simulink model "Experiment4_DOB_model2"  (R2012b)
settings: Solver=ode3  SolverMode=SingleTasking  StartTime=0.0  StopTime=5  FixedStep=0.002  RelTol=1e-3
values from neighbouring files (symbols this model uses):
  exp_A_DOB = 1    [model_DOB.mat]
  exp_model = 1    [model_ref.mat]
  exp_model_input = 1    [model_input.mat]
undefined symbols (not defined in the file or in its folder): K0, Kd, Ki, Kp, Plant_K, Plant_T1, Plant_T2, Q_T, T1, T2
libraries: simulink x4
settings Model: Creator=taoyi  LastModifiedBy=Administrator
settings DataIOCC: SignalLoggingSaveFormat=ModelDataLogs
settings OptimizationCC: BlockReduction=off  BooleanDataType=off
settings DebuggingCC: SaveWithParameterizedLinksMsg=none  SignalResolutionControl=TryResolveAllWithWarning  SolverPrmCheckMsg=none  MultiTaskDSMMsg=warning  MultiTaskCondExecSysMsg=none  StrictBusMsg=None
settings HardwareCC: TargetUnknown=on
settings RTWCC: IncludeERTFirstTime=on

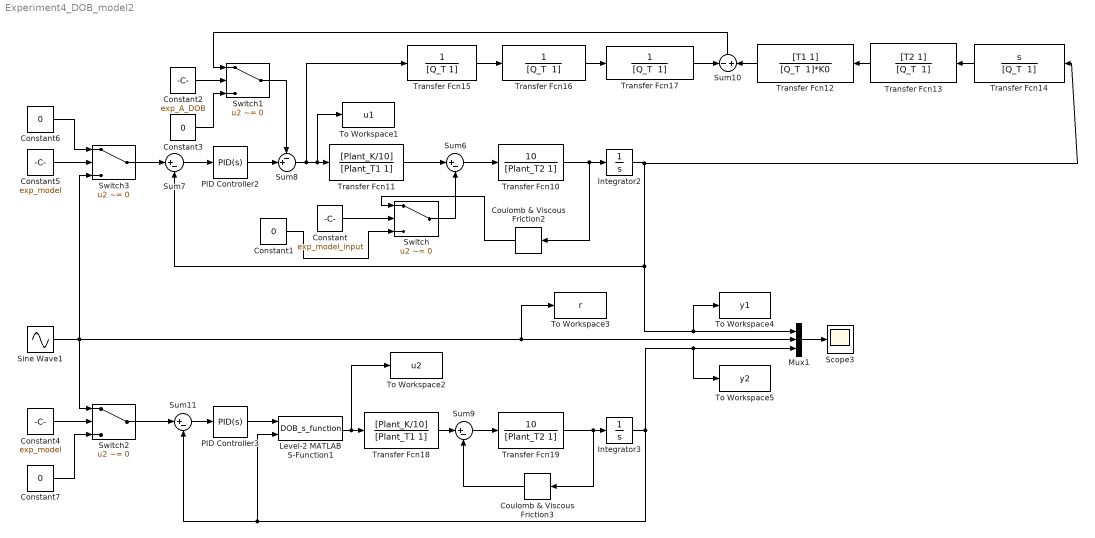
== system Experiment4_DOB_model2 ==
  Constant : Constant  Value=exp_model_input
  Constant{1,3,6..7} (4 alike) : Constant  Value=0
  Constant2 : Constant  Value=exp_A_DOB
  Constant4 : Constant  Value=exp_model
  Constant5 : Constant  Value=exp_model
  Coulomb & Viscous Friction2 : simulink/Discontinuities/Coulomb & Viscous Friction  offset=[20]  gain=0.3
  Coulomb & Viscous Friction3 : simulink/Discontinuities/Coulomb & Viscous Friction  offset=[20]  gain=0.3
  Integrator2 : Integrator
  Integrator3 : Integrator
  Level-2 MATLAB S-Function1 : M-S-Function  FunctionName=DOB_s_function  Parameters=K0,T1,T2,Q_T
  Mux1 : Mux  Inputs=3
  PID Controller2 : simulink/Continuous/PID Controller  Controller=PID  TimeDomain=Continuous-time  SampleTime=1  IntegratorMethod=Forward Euler  FilterMethod=Forward Euler  Form=Parallel  P=Kp  I=Ki  D=Kd  N=100  InitialConditionSource=internal  InitialConditionForIntegrator=0  InitialConditionForFilter=0  ExternalReset=none  LimitOutput=off  UpperSaturationLimit=inf  LowerSaturationLimit=-inf  LinearizeAsGain=on  AntiWindupMode=none  Kb=1  TrackingMode=off  Kt=1  PParamMin=[]  PParamMax=[]  IParamMin=[]  IParamMax=[]  DParamMin=[]  DParamMax=[]  NParamMin=[]  NParamMax=[]  KbParamMin=[]  KbParamMax=[]  KtParamMin=[]  KtParamMax=[]  POutMin=[]  POutMax=[]  IOutMin=[]  IOutMax=[]  DOutMin=[]  DOutMax=[]  NOutMin=[]  NOutMax=[]  KbOutMin=[]  KbOutMax=[]  KtOutMin=[]  KtOutMax=[]  IntegratorOutMin=[]  IntegratorOutMax=[]  FilterOutMin=[]  FilterOutMax=[]  SumOutMin=[]  SumOutMax=[]  SumI1OutMin=[]  SumI1OutMax=[]  SumI2OutMin=[]  SumI2OutMax=[]  SumI3OutMin=[]  SumI3OutMax=[]  SumDOutMin=[]  SumDOutMax=[]  SaturationOutMin=[]  SaturationOutMax=[]  IntegratorContinuousStateAttributes=''  IntegratorStateMustResolveToSignalObject=off  IntegratorRTWStateStorageClass=Auto  FilterContinuousStateAttributes=''  FilterStateMustResolveToSignalObject=off  FilterRTWStateStorageClass=Auto
  PID Controller3 : simulink/Continuous/PID Controller  Controller=PID  TimeDomain=Continuous-time  SampleTime=1  IntegratorMethod=Forward Euler  FilterMethod=Forward Euler  Form=Parallel  P=Kp  I=Ki  D=Kd  N=100  InitialConditionSource=internal  InitialConditionForIntegrator=0  InitialConditionForFilter=0  ExternalReset=none  LimitOutput=off  UpperSaturationLimit=inf  LowerSaturationLimit=-inf  LinearizeAsGain=on  AntiWindupMode=none  Kb=1  TrackingMode=off  Kt=1  PParamMin=[]  PParamMax=[]  IParamMin=[]  IParamMax=[]  DParamMin=[]  DParamMax=[]  NParamMin=[]  NParamMax=[]  KbParamMin=[]  KbParamMax=[]  KtParamMin=[]  KtParamMax=[]  POutMin=[]  POutMax=[]  IOutMin=[]  IOutMax=[]  DOutMin=[]  DOutMax=[]  NOutMin=[]  NOutMax=[]  KbOutMin=[]  KbOutMax=[]  KtOutMin=[]  KtOutMax=[]  IntegratorOutMin=[]  IntegratorOutMax=[]  FilterOutMin=[]  FilterOutMax=[]  SumOutMin=[]  SumOutMax=[]  SumI1OutMin=[]  SumI1OutMax=[]  SumI2OutMin=[]  SumI2OutMax=[]  SumI3OutMin=[]  SumI3OutMax=[]  SumDOutMin=[]  SumDOutMax=[]  SaturationOutMin=[]  SaturationOutMax=[]  IntegratorContinuousStateAttributes=''  IntegratorStateMustResolveToSignalObject=off  IntegratorRTWStateStorageClass=Auto  FilterContinuousStateAttributes=''  FilterStateMustResolveToSignalObject=off  FilterRTWStateStorageClass=Auto
  Scope3 : Scope
      settings: YMin=-25  YMax=27.5
  Sine Wave1 : Sin  Amplitude=20  Frequency=2*pi  SampleTime=0
  Sum10 : Sum  Inputs=-+
  Sum{6..7,9,11} (4 alike) : Sum  Inputs=|+-
  Sum8 : Sum  Inputs=-+|
  Switch{,1..3} (4 alike) : Switch  Criteria=u2 ~= 0
  To Workspace1 : ToWorkspace  VariableName=u1  SampleTime=-1
  To Workspace2 : ToWorkspace  VariableName=u2  SampleTime=-1
  To Workspace3 : ToWorkspace  VariableName=r  SampleTime=-1
  To Workspace4 : ToWorkspace  VariableName=y1  SampleTime=-1
  To Workspace5 : ToWorkspace  VariableName=y2  SampleTime=-1
  Transfer Fcn10 : TransferFcn  Numerator=[10]  Denominator=[Plant_T2 1]
  Transfer Fcn11 : TransferFcn  Numerator=[Plant_K/10]  Denominator=[Plant_T1 1]
  Transfer Fcn12 : TransferFcn  Numerator=[T1 1]  Denominator="[Q_T  1]*K0"
  Transfer Fcn13 : TransferFcn  Numerator=[T2 1]  Denominator="[Q_T  1]"
  Transfer Fcn14 : TransferFcn  Numerator=[1 0]  Denominator="[Q_T  1]"
  Transfer Fcn15 : TransferFcn  Denominator=[Q_T 1]
  Transfer Fcn16 : TransferFcn  Denominator="[Q_T  1]"
  Transfer Fcn17 : TransferFcn  Denominator="[Q_T  1]"
  Transfer Fcn18 : TransferFcn  Numerator=[Plant_K/10]  Denominator=[Plant_T1 1]
  Transfer Fcn19 : TransferFcn  Numerator=[10]  Denominator=[Plant_T2 1]
  wires:
  Transfer Fcn13/1 -> Transfer Fcn12/1
  Sum10/1 -> Switch1/1
  Transfer Fcn14/1 -> Transfer Fcn13/1
  Transfer Fcn17/1 -> Sum10/1
  Coulomb & Viscous Friction2/1 -> Switch/1
  Sum6/1 -> Transfer Fcn10/1
  Sum8/1 -> To Workspace1/1, Transfer Fcn11/1, Transfer Fcn15/1
  Transfer Fcn15/1 -> Transfer Fcn16/1
  PID Controller2/1 -> Sum8/2
  Transfer Fcn16/1 -> Transfer Fcn17/1
  Transfer Fcn12/1 -> Sum10/2
  Sum7/1 -> PID Controller2/1
  Transfer Fcn10/1 -> Coulomb & Viscous Friction2/1, Integrator2/1
  Transfer Fcn11/1 -> Sum6/1
  Sine Wave1/1 -> To Workspace3/1, Mux1/2, Switch3/3, Switch2/1
  Transfer Fcn18/1 -> Sum9/1
  Integrator3/1 -> To Workspace5/1, Mux1/3, Level-2 MATLAB S-Function1/2, Sum11/2
  Transfer Fcn19/1 -> Coulomb & Viscous Friction3/1, Integrator3/1
  Sum11/1 -> PID Controller3/1
  PID Controller3/1 -> Level-2 MATLAB S-Function1/1
  Coulomb & Viscous Friction3/1 -> Sum9/2
  Sum9/1 -> Transfer Fcn19/1
  Level-2 MATLAB S-Function1/1 -> To Workspace2/1, Transfer Fcn18/1
  Mux1/1 -> Scope3/1
  Integrator2/1 -> Transfer Fcn14/1, Sum7/2, To Workspace4/1, Mux1/1
  Switch/1 -> Sum6/2
  Constant1/1 -> Switch/3
  Constant/1 -> Switch/2
  Switch1/1 -> Sum8/1
  Constant3/1 -> Switch1/3
  Constant2/1 -> Switch1/2
  Constant4/1 -> Switch2/2
  Switch2/1 -> Sum11/1
  Constant5/1 -> Switch3/2
  Switch3/1 -> Sum7/1
  Constant6/1 -> Switch3/1
  Constant7/1 -> Switch2/3
